simulink model "lateral_path_transformer_demo"  (R2019b)
settings: Solver=FixedStepDiscrete  StartTime=0.0  StopTime=40  FixedStep=0.01  RelTol=1e-3  EnableMultiTasking=on
undefined symbols (not defined in the file or in its folder): path_data_D
libraries: simulink x2
Description:
  | Counter Implemented in a C++ S-function
settings Model: ExtModeTrigMode=oneshot  ExtModeArmWhenConnect=off  ExtModeAutoUpdateStatusClock=off  Creator=The MathWorks, Inc.  LastModifiedBy=chr
settings DataIOCC: SaveFormat=Array
settings OptimizationCC: BlockReduction=off  BooleanDataType=off  ExpressionDepthLimit=2147483647  InitFltsAndDblsToZero=on  LifeSpan=inf
settings DebuggingCC: SaveWithParameterizedLinksMsg=none  SignalResolutionControl=TryResolveAllWithWarning  MultiTaskDSMMsg=warning  MultiTaskCondExecSysMsg=none  FcnCallInpInsideContextMsg=warning  StateNameClashWarn=warning  SFUnexpectedBacktrackingDiag=warning  SFNoUnconditionalDefaultTransitionDiag=warning  SFExecutionAtInitializationDiag=none  ArithmeticOperatorsInVariantConditions=warning
settings HardwareCC: ProdBitPerPointer=32  ProdBitPerSizeT=32  ProdBitPerPtrDiffT=32  ProdLargestAtomicFloat=None  ProdIntDivRoundTo=Undefined  ProdEndianess=Unspecified  ProdWordSize=32  ProdHWDeviceType=32-bit Generic
settings ModelReferenceCC: PropagateSignalLabelsOutOfModel=off
settings SFSimCC: SimUseLocalCustomCode=off  CustomCodeUndefinedFunction=UseInterfaceOnly
settings RTWCC: Description=Generic Real-Time Target  RetainRTWFile=on  RTWUseLocalCustomCode=off
settings CodeAppCC: StateflowObjectComments=on
settings GRTTargetCC: TargetFcnLib=ansi_tfl_tmw.mat  TargetLangStandard=C89/C90 (ANSI)  GeneratePreprocessorConditionals=Disable all  CombineOutputUpdateFcns=off  GRTInterface=on
settings ConfigComp: CovMetricSettings=dw  CovHtmlReporting=on  CovSaveCumulativeToWorkspaceVar=on  CovSaveSingleToWorkspaceVar=on  CovExternalEMLEnable=off

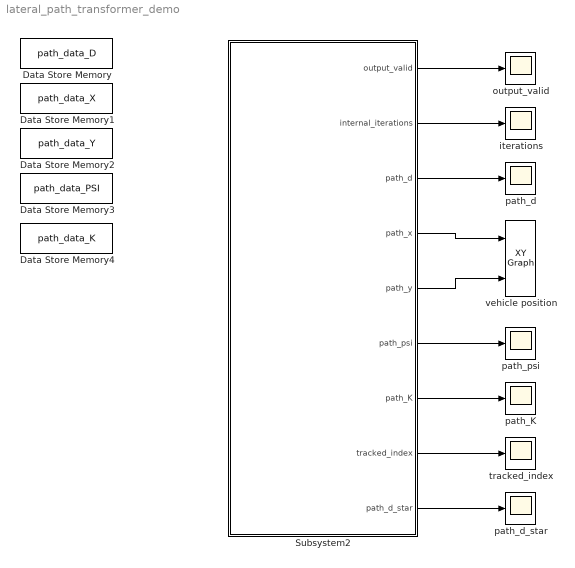
== system lateral_path_transformer_demo ==
  Data Store Memory : DataStoreMemory  DataStoreName=path_data_D  ReadBeforeWriteMsg=warning  WriteAfterWriteMsg=warning  WriteAfterReadMsg=warning  InitialValue=path_data.D  ShowAdditionalParam=off
  Data Store Memory1 : DataStoreMemory  DataStoreName=path_data_X  ReadBeforeWriteMsg=warning  WriteAfterWriteMsg=warning  WriteAfterReadMsg=warning  InitialValue=path_data.X  ShowAdditionalParam=off
  Data Store Memory2 : DataStoreMemory  DataStoreName=path_data_Y  ReadBeforeWriteMsg=warning  WriteAfterWriteMsg=warning  WriteAfterReadMsg=warning  InitialValue=path_data.Y  ShowAdditionalParam=off
  Data Store Memory3 : DataStoreMemory  DataStoreName=path_data_PSI  ReadBeforeWriteMsg=warning  WriteAfterWriteMsg=warning  WriteAfterReadMsg=warning  InitialValue=path_data.PSI  ShowAdditionalParam=off
  Data Store Memory4 : DataStoreMemory  DataStoreName=path_data_K  ReadBeforeWriteMsg=warning  WriteAfterWriteMsg=warning  WriteAfterReadMsg=warning  InitialValue=path_data.K  ShowAdditionalParam=off
  Subsystem2 : Subsystem
  iterations : Scope
  output_valid : Scope
  path_K : Scope
  path_d : Scope
  path_d_star : Scope
  path_psi : Scope
  tracked_index : Scope
  vehicle position : simulink/Sinks/XY Graph  xmin=-40  xmax=40  ymin=-40  ymax=40  st=-1
  wires:
  Subsystem2/1(output_valid) -> output_valid/1
  Subsystem2/2(internal_iterations) -> iterations/1
  Subsystem2/3(path_d) -> path_d/1
  Subsystem2/6(path_psi) -> path_psi/1
  Subsystem2/4(path_x) -> vehicle position/1
  Subsystem2/5(path_y) -> vehicle position/2
  Subsystem2/7(path_K) -> path_K/1
  Subsystem2/8(tracked_index) -> tracked_index/1
  Subsystem2/9(path_d_star) -> path_d_star/1

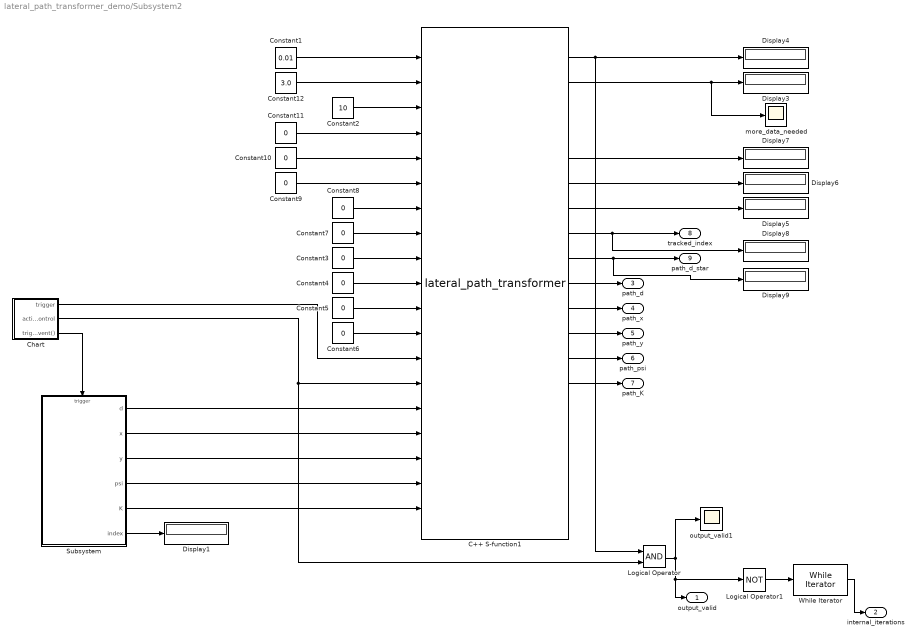
== system lateral_path_transformer_demo/Subsystem2 ==
  C++ S-function1 : S-Function  FunctionName=lateral_path_transformer  Parameters=-1  SFunctionDeploymentMode=off  EnableBusSupport=off
      mask Display:
      | % copy and paste these commands into the field 'icon drawing commands' of the block mask:
      | % right-click on block -> 'Mask' -> 'Edit Mask' -> 'Mask Editor' -> 'Icons & Ports'
      | 
      | port_label('input', 1, 'Ts')
      | port_label('input', 2, 'wheelbase')
      | port_label('input', 3, 'velocity_')
      | port_label('input', 4, 'Delta_l_r')
      | port_label('input', 5, 'Delta_l_r_dot')
      | port_label('input', 6, 'Delta_l_r_dotdot')
      | port_label('input', 7, 'd0')
      | port_label('input', 8, 'x0')
      | port_label('input', 9, 'y0')
      | port_label('input', 10, 'psi0')
      | port_label('input', 11, 'delta0')
      | port_label('input', 12, 'delta_dot0')
      | port_label('input', 13, 'async_input_data_valid')
      | port_label('input', 14, 'input_sample_valid')
      | port_label('input', 15, 'd_sample')
      | port_label('input', 16, 'x_sample')
      | port_label('input', 17, 'y_sample')
      | port_label('input', 18, 'psi_sample')
      | port_label('input', 19, 'K_sample')
      | port_label('output', 1, 'output_valid')
      | port_label('output', 2, 'need_more_path_input_data')
      | port_label('output', 3, 'distance_at_the_end_of_horizon')
      | port_label('output', 4, 'distance_ahead')
      | port_label('output', 5, 'head_index')
      | port_label('output', 6, 'read_position')
      | port_label('output', 7, 'elements_free_to_write')
      | port_label('output', 8, 'tracked_index')
      | port_label('output', 9, 'path_d_star')
      | port_label('output', 10, 'path_d')
      | port_label('output', 11, 'path_x')
      | port_label('output', 12, 'path_y')
      | port_label('output', 13, 'path_psi')
      | port_label('output', 14, 'path_K')
      | port_label('output', 15, 'vehicle_delta')
      | port_label('output', 16, 'vehicle_delta_dot')
      | port_label('output', 17, 'vehicle_psi')
      | port_label('output', 18, 'vehicle_psi_dot')
      | port_label('output', 19, 'velocity')
  Chart : Stateflow chart  BlockKeywords=__PRM__SERIALIZED__DATA__:Stateflow Chart,Stateflow Diagram  TreatAsAtomicUnit=on
  Constant1 : Constant  Value=0.01
  Constant{3..11} (9 alike) : Constant  Value=0
  Constant12 : Constant  Value=3.0
  Constant2 : Constant  Value=10
  Display{1,3..9} (8 alike) : Display
  Logical Operator : Logic  AllPortsSameDT=off  OutDataTypeStr=boolean
  Logical Operator1 : Logic  Operator=NOT  AllPortsSameDT=off  OutDataTypeStr=boolean
  Subsystem : Subsystem
  While Iterator : WhileIterator  MaxIters=1000  WhileBlockType=do-while  ShowIterationPort=on
  more_data_needed : Scope
  output_valid1 : Scope
  output_valid : Outport
  internal_iterations : Outport  Port=2
  path_d : Outport  Port=3
  path_x : Outport  Port=4
  path_y : Outport  Port=5
  path_psi : Outport  Port=6
  path_K : Outport  Port=7
  tracked_index : Outport  Port=8
  path_d_star : Outport  Port=9
  wires:
  C++ S-function1/6 -> Display6/1
  Constant4/1 -> C++ S-function1/10
  Constant7/1 -> C++ S-function1/8
  Subsystem/6(index) -> Display1/1
  Constant6/1 -> C++ S-function1/12
  C++ S-function1/8 -> tracked_index/1, Display8/1
  Constant3/1 -> C++ S-function1/9
  Constant10/1 -> C++ S-function1/5
  Subsystem/3(y) -> C++ S-function1/17
  Constant2/1 -> C++ S-function1/3
  Chart/3(trigger_event()) -> Subsystem/Trigger
  Subsystem/4(psi) -> C++ S-function1/18
  Subsystem/2(x) -> C++ S-function1/16
  Constant11/1 -> C++ S-function1/4
  C++ S-function1/2 -> more_data_needed/1, Display3/1
  Logical Operator/1 -> output_valid/1, Logical Operator1/1, output_valid1/1
  C++ S-function1/9 -> Display9/1, path_d_star/1
  Constant5/1 -> C++ S-function1/11
  Subsystem/5(K) -> C++ S-function1/19
  Chart/2(activate_control) -> Logical Operator/2, C++ S-function1/14
  C++ S-function1/7 -> Display5/1
  Constant9/1 -> C++ S-function1/6
  C++ S-function1/1 -> Logical Operator/1, Display4/1
  Chart/1(trigger) -> C++ S-function1/13
  Constant8/1 -> C++ S-function1/7
  C++ S-function1/5 -> Display7/1
  Subsystem/1(d) -> C++ S-function1/15
  Logical Operator1/1 -> While Iterator/1
  While Iterator/1 -> internal_iterations/1
  C++ S-function1/10 -> path_d/1
  C++ S-function1/11 -> path_x/1
  C++ S-function1/12 -> path_y/1
  C++ S-function1/13 -> path_psi/1
  C++ S-function1/14 -> path_K/1
  Constant1/1 -> C++ S-function1/1
  Constant12/1 -> C++ S-function1/2

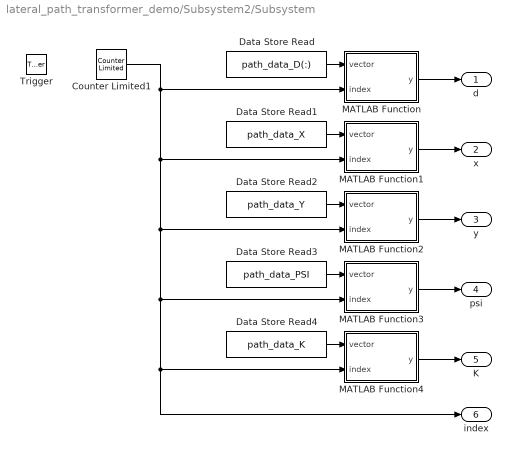
== system lateral_path_transformer_demo/Subsystem2/Subsystem ==
  Trigger : TriggerPort  TriggerType=function-call  VariantControl=Variant  PortDimensions=1
  Counter Limited1 : simulink/Sources/Counter Limited  uplimit=path_data.N - 1  tsamp=-1
  Data Store Read : DataStoreRead  DataStoreName=path_data_D  DataStoreElements=path_data_D(:)
  Data Store Read1 : DataStoreRead  DataStoreName=path_data_X
  Data Store Read2 : DataStoreRead  DataStoreName=path_data_Y
  Data Store Read3 : DataStoreRead  DataStoreName=path_data_PSI
  Data Store Read4 : DataStoreRead  DataStoreName=path_data_K
  MATLAB Function : MATLAB Function  TreatAsAtomicUnit=on
  MATLAB Function1 : MATLAB Function  TreatAsAtomicUnit=on
  MATLAB Function2 : MATLAB Function  TreatAsAtomicUnit=on
  MATLAB Function3 : MATLAB Function  TreatAsAtomicUnit=on
  MATLAB Function4 : MATLAB Function  TreatAsAtomicUnit=on
  d : Outport
  x : Outport  Port=2
  y : Outport  Port=3
  psi : Outport  Port=4
  K : Outport  Port=5
  index : Outport  Port=6
  wires:
  Data Store Read/1 -> MATLAB Function/1(vector)
  MATLAB Function/1(y) -> d/1
  MATLAB Function1/1(y) -> x/1
  Data Store Read1/1 -> MATLAB Function1/1(vector)
  MATLAB Function2/1(y) -> y/1
  Data Store Read2/1 -> MATLAB Function2/1(vector)
  MATLAB Function3/1(y) -> psi/1
  Data Store Read3/1 -> MATLAB Function3/1(vector)
  Counter Limited1/1 -> index/1, MATLAB Function4/2(index), MATLAB Function3/2(index), MATLAB Function2/2(index), MATLAB Function1/2(index), MATLAB Function/2(index)
  MATLAB Function4/1(y) -> K/1
  Data Store Read4/1 -> MATLAB Function4/1(vector)

== matlab function lateral_path_transformer_demo/Subsystem2/Subsystem/MATLAB Function ==
  data: vector input; y output; index input
function y = fcn(vector, index)

y = vector(index+1);

== matlab function lateral_path_transformer_demo/Subsystem2/Subsystem/MATLAB Function1 ==
  data: vector input; y output; index input
function y = fcn(vector, index)

y = vector(index+1);

== stateflow chart lateral_path_transformer_demo/Subsystem2/Chart ==
  state init
    trigger=false;
    activate_control=false;
  state fill_buffer
    bind: trigger_event;
    en, du: trigger_event;
    trigger=true;
    activate_control=false;
  state buffer_filled
    trigger=false;
    activate_control=true;
  (default) -> init
  init -> fill_buffer : after(2, tick)
  buffer_filled -> fill_buffer : after(100,tick)
  fill_buffer -> buffer_filled : after(200, tick)
  data: trigger output boolean; activate_control output boolean
  events: trigger_event output FUNCTION_CALL_EVENT

== matlab function lateral_path_transformer_demo/Subsystem2/Subsystem/MATLAB Function2 ==
  data: vector input; y output; index input
function y = fcn(vector, index)

y = vector(index+1);

== matlab function lateral_path_transformer_demo/Subsystem2/Subsystem/MATLAB Function3 ==
  data: vector input; y output; index input
function y = fcn(vector, index)

y = vector(index+1);

== matlab function lateral_path_transformer_demo/Subsystem2/Subsystem/MATLAB Function4 ==
  data: vector input; y output; index input
function y = fcn(vector, index)

y = vector(index+1);
